simulink library "momentum_dump_lib"  (R2016b)
settings: Solver=VariableStepAuto  StartTime=0.0  StopTime=10.0  RelTol=1e-3
undefined symbols (not defined in the file or in its folder): fsw_params
libraries: vrlib x1, dspmathops x1
settings Model: Creator=unsik  LastModifiedBy=evich

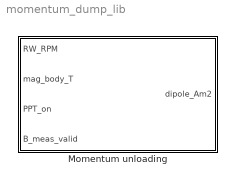
== system momentum_dump_lib ==
  Momentum unloading : Subsystem

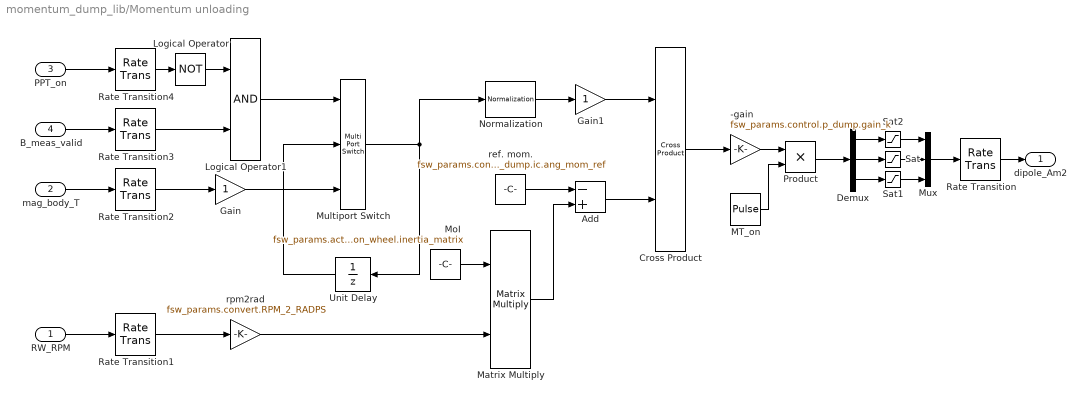
== system momentum_dump_lib/Momentum unloading ==
  RW_RPM : Inport
  mag_body_T : Inport  Port=2
  PPT_on : Inport  Port=3
  B_meas_valid : Inport  Port=4
  -gain : Gain  Gain=fsw_params.control.p_dump.gain_k
  Add : Sum  Inputs=-+
  Cross Product : vrlib/Utilities/Cross Product
  Demux : Demux  Outputs=3
  Gain : Gain
  Gain1 : Gain
  Logical Operator : Logic  Operator=NOT  AllPortsSameDT=off  OutDataTypeStr=boolean
  Logical Operator1 : Logic  AllPortsSameDT=off  OutDataTypeStr=boolean
  MT_on : DiscretePulseGenerator  PulseType=Time based  Period=1  PulseWidth=fsw_params.actuators.magnetorquer.actuation_time_pct
  Matrix Multiply : Product  Inputs=**  Multiplication=Matrix(*)
  MoI : Constant  Value=fsw_params.actuators.reaction_wheel.inertia_matrix
  Multiport Switch : MultiPortSwitch  DataPortOrder=Zero-based contiguous  Inputs=2
  Mux : Mux  Inputs=3
  Normalization : dspmathops/Normalization  NormType=Squared 2-norm  Bias=1e-10  NormOver=Each column  Dimension=1  outputDataTypeStr=Inherit: Same as product output  outputLastDataTypeStr=Inherit: Same as product output  outputMin=[]  outputMax=[]  accumDataTypeStr=Inherit: Same as product output  accumLastDataTypeStr=Inherit: Same as product output  roundingMode=Floor  overflowMode=off
  Product : Product
  Rate Transition : RateTransition  X0=fsw_params.control.p_dump.ic.rt_dipole_Am2
  Rate Transition1 : RateTransition  X0=fsw_params.control.p_dump.ic.rt_rw_RPM  OutPortSampleTime=fsw_params.control.p_dump.sample_time_s
  Rate Transition2 : RateTransition  X0=fsw_params.control.p_dump.ic.rt_mag_body_T  OutPortSampleTime=fsw_params.control.p_dump.sample_time_s
  Rate Transition3 : RateTransition  X0=fsw_params.control.p_dump.ic.rt_B_meas_valid  OutPortSampleTime=fsw_params.control.p_dump.sample_time_s
  Rate Transition4 : RateTransition  X0=fsw_params.control.p_dump.ic.rt_PPT_on  OutPortSampleTime=fsw_params.control.p_dump.sample_time_s
  Sat : Saturate  UpperLimit=fsw_params.actuators.magnetorquer.max_dipole_y  LowerLimit=-fsw_params.actuators.magnetorquer.max_dipole_y
  Sat1 : Saturate  UpperLimit=fsw_params.actuators.magnetorquer.max_dipole_z  LowerLimit=-fsw_params.actuators.magnetorquer.max_dipole_z
  Sat2 : Saturate  UpperLimit=fsw_params.actuators.magnetorquer.max_dipole_x  LowerLimit=-fsw_params.actuators.magnetorquer.max_dipole_x
  Unit Delay : UnitDelay  InitialCondition=fsw_params.control.p_dump.ic.rt_mag_body_T  SampleTime=-1
  ref. mom. : Constant  Value=fsw_params.control.p_dump.ic.ang_mom_ref
  rpm2rad : Gain  Gain=fsw_params.convert.RPM_2_RADPS
  dipole_Am2 : Outport
  wires:
  ref. mom./1 -> Add/1
  Matrix Multiply/1 -> Add/2
  MoI/1 -> Matrix Multiply/1
  Multiport Switch/1 -> Normalization/1, Unit Delay/1
  rpm2rad/1 -> Matrix Multiply/2
  Add/1 -> Cross Product/2
  Cross Product/1 -> -gain/1
  Logical Operator1/1 -> Multiport Switch/1
  Logical Operator/1 -> Logical Operator1/1
  Rate Transition3/1 -> Logical Operator1/2
  Rate Transition4/1 -> Logical Operator/1
  Rate Transition2/1 -> Gain/1
  Unit Delay/1 -> Multiport Switch/2
  PPT_on/1 -> Rate Transition4/1
  B_meas_valid/1 -> Rate Transition3/1
  mag_body_T/1 -> Rate Transition2/1
  RW_RPM/1 -> Rate Transition1/1
  Rate Transition1/1 -> rpm2rad/1
  Demux/2 -> Sat/1
  Demux/1 -> Sat2/1
  Demux/3 -> Sat1/1
  Sat1/1 -> Mux/3
  Sat/1 -> Mux/2
  Sat2/1 -> Mux/1
  Mux/1 -> Rate Transition/1
  Gain/1 -> Multiport Switch/3
  Gain1/1 -> Cross Product/1
  Normalization/1 -> Gain1/1
  Rate Transition/1 -> dipole_Am2/1
  -gain/1 -> Product/1
  Product/1 -> Demux/1
  MT_on/1 -> Product/2
